simulink subsystem "Subsystem_Driver_Battery_BAv02"  (R2022b)
settings: Solver=VariableStepAuto  StartTime=0.0  StopTime=10.0  RelTol=1e-3
undefined symbols (not defined in the file): driver, param, route, weatherSim
libraries: slpidlib x3
settings Model: Creator=giaco  LastModifiedBy=giaco

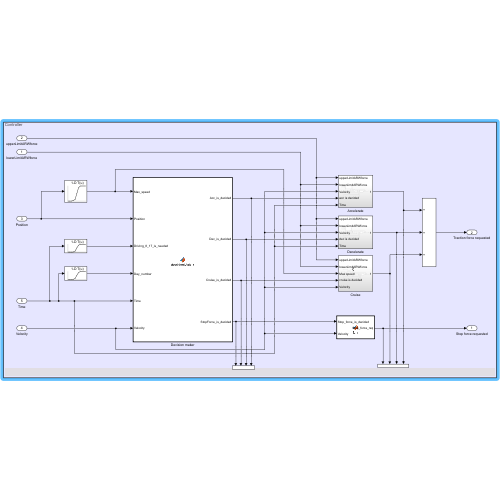
[thumbnail: Simulink's stored preview of the top-level diagram]
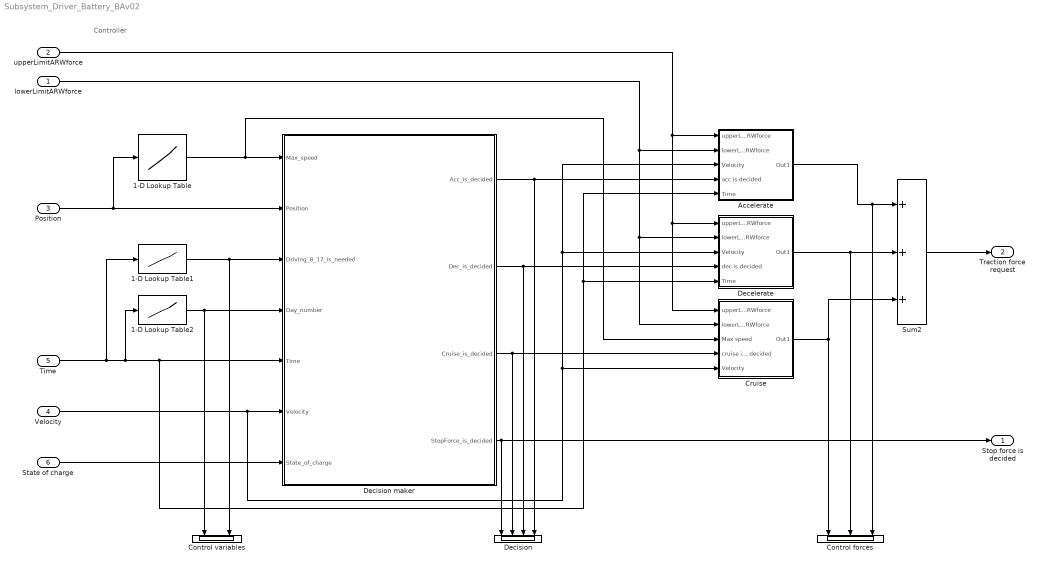
== system Subsystem_Driver_Battery_BAv02 ==
  note: Controller
  lowerLimitARWforce : Inport
  upperLimitARWforce : Inport  Port=2
  Position : Inport  Port=3
  Velocity : Inport  Port=4
  Time : Inport  Port=5
  State of charge : Inport  Port=6
  1-D Lookup Table : Lookup_n-D  NumberOfTableDimensions=1  BreakpointsForDimension1=route.dist  Table=route.maxSpeed  InternalRulePriority=Speed  RndMeth=Simplest
  1-D Lookup Table1 : Lookup_n-D  NumberOfTableDimensions=1  BreakpointsForDimension1=weatherSim.irradiance.timeSec  Table=weatherSim.irradiance.driving_8_17_Sec  InternalRulePriority=Speed
  1-D Lookup Table2 : Lookup_n-D  NumberOfTableDimensions=1  BreakpointsForDimension1=weatherSim.irradiance.timeSec  Table=weatherSim.irradiance.dayNumSec  InternalRulePriority=Speed
  Accelerate : Subsystem
  Control forces : Scope  NumInputPorts=3
  Control variables : Scope  NumInputPorts=2
  Cruise : Subsystem
  Decelerate : Subsystem
  Decision : Scope  NumInputPorts=4
  Decision maker : MATLAB Function  TreatAsAtomicUnit=on
  Sum2 : Sum  Inputs=+++
  Stop force is decided : Outport
  Traction force request : Outport  Port=2
  wires:
  Decision maker/4(StopForce_is_decided) -> Stop force is decided/1, Decision/1
  Accelerate/1(Out1) -> Control forces/3, Sum2/1
  upperLimitARWforce/1 -> Decelerate/1(upperLimitARWforce), Cruise/1(upperLimitARWforce), Accelerate/1(upperLimitARWforce)
  Sum2/1 -> Traction force request/1
  Velocity/1 -> Decision maker/6(Velocity), Accelerate/3(Velocity), Decelerate/3(Velocity), Cruise/5(Velocity)
  Decision maker/2(Dec_is_decided) -> Decision/3, Decelerate/4(dec is decided)
  Decision maker/1(Acc_is_decided) -> Accelerate/4(acc is decided), Decision/4
  lowerLimitARWforce/1 -> Accelerate/2(lowerLimitARWforce), Decelerate/2(lowerLimitARWforce), Cruise/2(lowerLimitARWforce)
  1-D Lookup Table/1 -> Decision maker/1(Max_speed), Cruise/3(Max speed)
  Decelerate/1(Out1) -> Control forces/2, Sum2/2
  Time/1 -> 1-D Lookup Table1/1, 1-D Lookup Table2/1, Decision maker/5(Time), Accelerate/5(Time), Decelerate/5(Time)
  Decision maker/3(Cruise_is_decided) -> Decision/2, Cruise/4(cruise is decided)
  Cruise/1(Out1) -> Control forces/1, Sum2/3
  Position/1 -> Decision maker/2(Position), 1-D Lookup Table/1
  1-D Lookup Table1/1 -> Control variables/2, Decision maker/3(Driving_8_17_is_needed)
  1-D Lookup Table2/1 -> Control variables/1, Decision maker/4(Day_number)
  State of charge/1 -> Decision maker/7(State_of_charge)

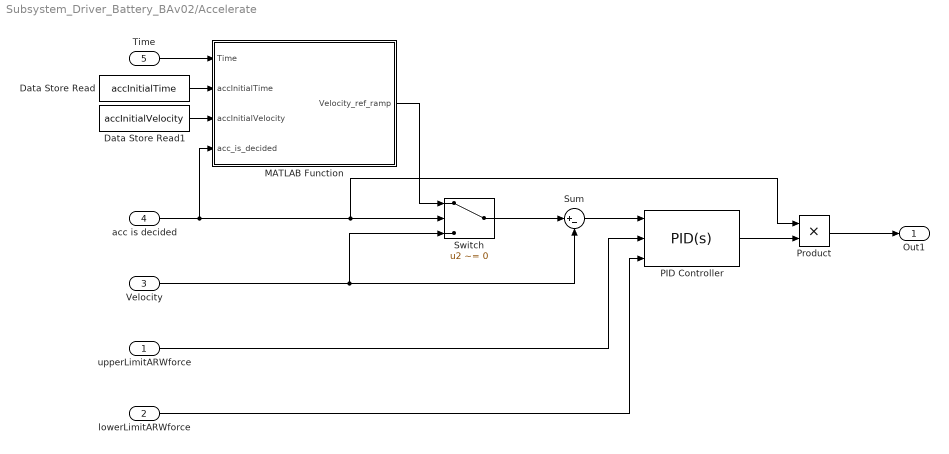
== system Subsystem_Driver_Battery_BAv02/Accelerate ==
  upperLimitARWforce : Inport
  lowerLimitARWforce : Inport  Port=2
  Velocity : Inport  Port=3
  acc is decided : Inport  Port=4
  Time : Inport  Port=5
  Data Store Read : DataStoreRead  DataStoreName=accInitialTime  IndexOptions=Index vector (dialog)  Indices=1  OutputSizes=1
  Data Store Read1 : DataStoreRead  DataStoreName=accInitialVelocity  IndexOptions=Index vector (dialog)  Indices=1  OutputSizes=1
  MATLAB Function : MATLAB Function  TreatAsAtomicUnit=on
  PID Controller : slpidlib/PID Controller  Controller=PID  Form=Ideal  TimeDomain=Continuous-time  UseExternalTs=off  SampleTime=-1  IntegratorMethod=Forward Euler  FilterMethod=Forward Euler  ControllerParametersSource=internal  P=4000  I=80/1  UseKiTs=off  D=0  N=100  UseFilter=on  TunerSelectOption=Transfer Function Based (PID Tuner App)  InitialConditionSource=internal  InitialConditionForIntegrator=0  InitialConditionForFilter=0  DifferentiatorICPrevScaledInput=0  ExternalReset=none  TrackingMode=off  Kt=1  LimitOutput=on  SatLimitsSource=external  UpperSaturationLimit=param.motor.maxTorque * param.motor.transmissionRatio / param.suspension.rWheel  LowerSaturationLimit=param.motor.minTorque * param.motor.transmissionRatio / param.suspension.rWheel  LinearizeAsGain=on  AntiWindupMode=none  Kb=1  LimitIntegrator=off  UpperIntegratorSaturationLimit=inf  LowerIntegratorSaturationLimit=-inf  POutMin=[]  POutMax=[]  IOutMin=[]  IOutMax=[]  DOutMin=[]  DOutMax=[]  NOutMin=[]  NOutMax=[]  SumOutMin=[]  SumOutMax=[]  SaturationOutMin=[]  SaturationOutMax=[]  PParamMin=[]  PParamMax=[]  IParamMin=[]  IParamMax=[]  DParamMin=[]  DParamMax=[]  NParamMin=[]  NParamMax=[]  KbParamMin=[]  KbParamMax=[]  KtParamMin=[]  KtParamMax=[]  KbOutMin=[]  KbOutMax=[]  KtOutMin=[]  KtOutMax=[]  IntegratorOutMin=[]  IntegratorOutMax=[]  FilterOutMin=[]  FilterOutMax=[]  SumI1OutMin=[]  SumI1OutMax=[]  SumI2OutMin=[]  SumI2OutMax=[]  SumI3OutMin=[]  SumI3OutMax=[]  SumI4OutMin=[]  SumI4OutMax=[]  SumDOutMin=[]  SumDOutMax=[]  DifferentiatorOutMin=[]  DifferentiatorOutMax=[]  FilterDiffOutCoefMin=[]  FilterDiffOutCoefMax=[]  ReciprocalOutMin=[]  ReciprocalOutMax=[]  SumDenOutMin=[]  SumDenOutMax=[]  SumNumOutMin=[]  SumNumOutMax=[]  DivideOutMin=[]  DivideOutMax=[]  UdiffTsProdOutMin=[]  UdiffTsProdOutMax=[]  NTsProdOutMin=[]  NTsProdOutMax=[]  UintegralTsProdOutMin=[]  UintegralTsProdOutMax=[]  UngainTsProdOutMin=[]  UngainTsProdOutMax=[]  ClampingZeroOutDataTypeStr=Inherit: Inherit via back propagation  ClampingZeroOutMin=[]  ClampingZeroOutMax=[]  FilterDenConstantOutDataTypeStr=Inherit: Inherit via back propagation  FilterDenConstantOutMin=[]  FilterDenConstantOutMax=[]  PCopyOutDataTypeStr=Inherit: Inherit via back propagation  PCopyOutMin=[]  PCopyOutMax=[]  NCopyOutDataTypeStr=Inherit: Inherit via back propagation  NCopyOutMin=[]  NCopyOutMax=[]  IntegratorContinuousStateAttributes=''  IntegratorStateMustResolveToSignalObject=off  IntegratorRTWStateStorageClass=Auto  FilterContinuousStateAttributes=''  FilterStateMustResolveToSignalObject=off  FilterRTWStateStorageClass=Auto  ParallelPVariant=Passthrough  IdealPVariant=InternalParameters  IVariant=InternalParameters  DVariant=InternalParameters  IntegratorVariant=Continuous  SatVariant=External  AWVariant=Passthrough  PCopyVariant=Disabled  TRVariant=Disabled  FdbkBlocksVariant=Forward  IdealPFdbkVariant=Disabled  SatFdbkVariant=Disabled  DerivativeFilterVariant=ContFilter  NVariant=InternalParameters  NCopyVariant=Disabled  FilterICVariant=InternalICsFilter  IntegratorICVariant=InternalICs  ExternalResetVariant=Disabled  TRSumVariant=Passthrough  SumFdbkVariant=Disabled  SumVariant=Sum_PID  TsampFilterVariant=InternalTs  TsampNgainVariant=Passthrough  TsampIntegralVariant=Passthrough  ExternalSaturationOutDataTypeStr=Inherit: Same as second input
  Product : Product
  Sum : Sum  Inputs=|+-
  Switch : Switch  Criteria=u2 ~= 0  SaturateOnIntegerOverflow=off  InputSameDT=off
  Out1 : Outport
  wires:
  acc is decided/1 -> MATLAB Function/4(acc_is_decided), Product/1, Switch/2
  Switch/1 -> Sum/1
  Velocity/1 -> Sum/2, Switch/3
  Sum/1 -> PID Controller/1
  PID Controller/1 -> Product/2
  Product/1 -> Out1/1
  Time/1 -> MATLAB Function/1(Time)
  MATLAB Function/1(Velocity_ref_ramp) -> Switch/1
  Data Store Read/1 -> MATLAB Function/2(accInitialTime)
  Data Store Read1/1 -> MATLAB Function/3(accInitialVelocity)
  upperLimitARWforce/1 -> PID Controller/2
  lowerLimitARWforce/1 -> PID Controller/3

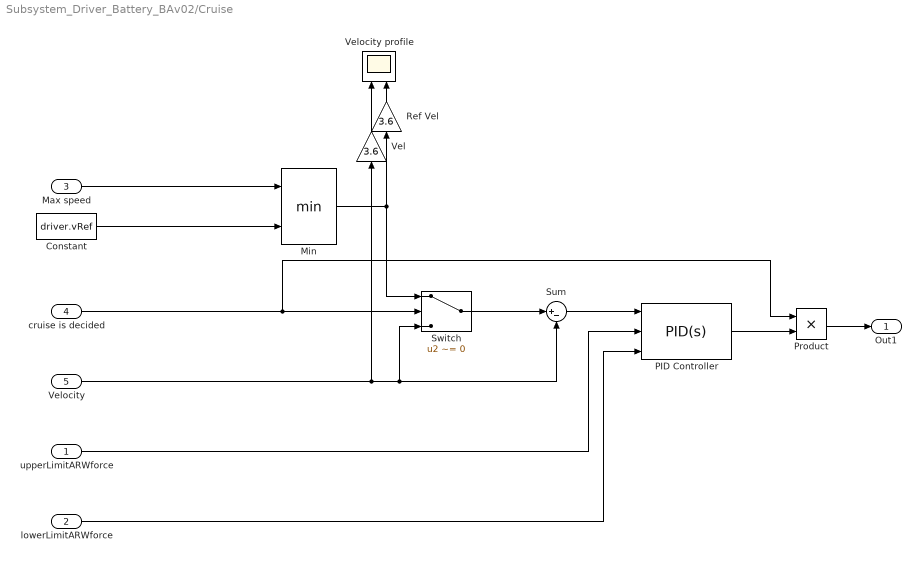
== system Subsystem_Driver_Battery_BAv02/Cruise ==
  upperLimitARWforce : Inport
  lowerLimitARWforce : Inport  Port=2
  Max speed : Inport  Port=3
  cruise is decided : Inport  Port=4
  Velocity : Inport  Port=5
  Constant : Constant  Value=driver.vRef
  Min : MinMax  Inputs=2
  PID Controller : slpidlib/PID Controller  Controller=PID  Form=Ideal  TimeDomain=Continuous-time  UseExternalTs=off  SampleTime=-1  IntegratorMethod=Forward Euler  FilterMethod=Forward Euler  ControllerParametersSource=internal  P=2000  I=1/500  UseKiTs=off  D=0  N=100  UseFilter=on  TunerSelectOption=Transfer Function Based (PID Tuner App)  InitialConditionSource=internal  InitialConditionForIntegrator=0  InitialConditionForFilter=0  DifferentiatorICPrevScaledInput=0  ExternalReset=none  TrackingMode=off  Kt=1  LimitOutput=on  SatLimitsSource=external  UpperSaturationLimit=param.motor.maxTorque * param.motor.transmissionRatio / param.suspension.rWheel  LowerSaturationLimit=param.motor.minTorque * param.motor.transmissionRatio / param.suspension.rWheel  LinearizeAsGain=on  AntiWindupMode=none  Kb=1  LimitIntegrator=off  UpperIntegratorSaturationLimit=inf  LowerIntegratorSaturationLimit=-inf  POutMin=[]  POutMax=[]  IOutMin=[]  IOutMax=[]  DOutMin=[]  DOutMax=[]  NOutMin=[]  NOutMax=[]  SumOutMin=[]  SumOutMax=[]  SaturationOutMin=[]  SaturationOutMax=[]  PParamMin=[]  PParamMax=[]  IParamMin=[]  IParamMax=[]  DParamMin=[]  DParamMax=[]  NParamMin=[]  NParamMax=[]  KbParamMin=[]  KbParamMax=[]  KtParamMin=[]  KtParamMax=[]  KbOutMin=[]  KbOutMax=[]  KtOutMin=[]  KtOutMax=[]  IntegratorOutMin=[]  IntegratorOutMax=[]  FilterOutMin=[]  FilterOutMax=[]  SumI1OutMin=[]  SumI1OutMax=[]  SumI2OutMin=[]  SumI2OutMax=[]  SumI3OutMin=[]  SumI3OutMax=[]  SumI4OutMin=[]  SumI4OutMax=[]  SumDOutMin=[]  SumDOutMax=[]  DifferentiatorOutMin=[]  DifferentiatorOutMax=[]  FilterDiffOutCoefMin=[]  FilterDiffOutCoefMax=[]  ReciprocalOutMin=[]  ReciprocalOutMax=[]  SumDenOutMin=[]  SumDenOutMax=[]  SumNumOutMin=[]  SumNumOutMax=[]  DivideOutMin=[]  DivideOutMax=[]  UdiffTsProdOutMin=[]  UdiffTsProdOutMax=[]  NTsProdOutMin=[]  NTsProdOutMax=[]  UintegralTsProdOutMin=[]  UintegralTsProdOutMax=[]  UngainTsProdOutMin=[]  UngainTsProdOutMax=[]  ClampingZeroOutDataTypeStr=Inherit: Inherit via back propagation  ClampingZeroOutMin=[]  ClampingZeroOutMax=[]  FilterDenConstantOutDataTypeStr=Inherit: Inherit via back propagation  FilterDenConstantOutMin=[]  FilterDenConstantOutMax=[]  PCopyOutDataTypeStr=Inherit: Inherit via back propagation  PCopyOutMin=[]  PCopyOutMax=[]  NCopyOutDataTypeStr=Inherit: Inherit via back propagation  NCopyOutMin=[]  NCopyOutMax=[]  IntegratorContinuousStateAttributes=''  IntegratorStateMustResolveToSignalObject=off  IntegratorRTWStateStorageClass=Auto  FilterContinuousStateAttributes=''  FilterStateMustResolveToSignalObject=off  FilterRTWStateStorageClass=Auto  ParallelPVariant=Passthrough  IdealPVariant=InternalParameters  IVariant=InternalParameters  DVariant=InternalParameters  IntegratorVariant=Continuous  SatVariant=External  AWVariant=Passthrough  PCopyVariant=Disabled  TRVariant=Disabled  FdbkBlocksVariant=Forward  IdealPFdbkVariant=Disabled  SatFdbkVariant=Disabled  DerivativeFilterVariant=ContFilter  NVariant=InternalParameters  NCopyVariant=Disabled  FilterICVariant=InternalICsFilter  IntegratorICVariant=InternalICs  ExternalResetVariant=Disabled  TRSumVariant=Passthrough  SumFdbkVariant=Disabled  SumVariant=Sum_PID  TsampFilterVariant=InternalTs  TsampNgainVariant=Passthrough  TsampIntegralVariant=Passthrough  ExternalSaturationOutDataTypeStr=Inherit: Same as second input
  Product : Product
  Ref Vel : Gain  Gain=3.6
  Sum : Sum  Inputs=|+-
  Switch : Switch  Criteria=u2 ~= 0  SaturateOnIntegerOverflow=off  InputSameDT=off
  Vel : Gain  Gain=3.6
  Velocity profile : Scope  NumInputPorts=2
  Out1 : Outport
  wires:
  cruise is decided/1 -> Product/1, Switch/2
  Max speed/1 -> Min/1
  Constant/1 -> Min/2
  Velocity/1 -> Vel/1, Switch/3, Sum/2
  Switch/1 -> Sum/1
  PID Controller/1 -> Product/2
  Sum/1 -> PID Controller/1
  Product/1 -> Out1/1
  lowerLimitARWforce/1 -> PID Controller/3
  upperLimitARWforce/1 -> PID Controller/2
  Ref Vel/1 -> Velocity profile/2
  Min/1 -> Switch/1, Ref Vel/1
  Vel/1 -> Velocity profile/1

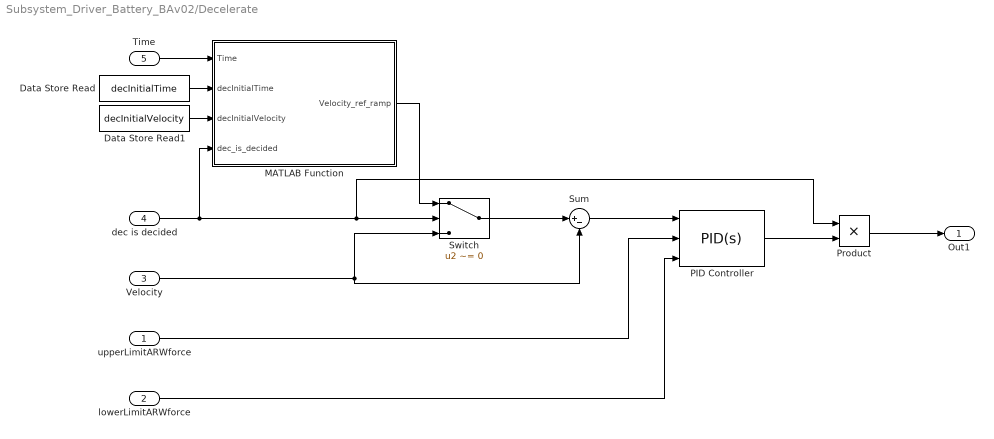
== system Subsystem_Driver_Battery_BAv02/Decelerate ==
  upperLimitARWforce : Inport
  lowerLimitARWforce : Inport  Port=2
  Velocity : Inport  Port=3
  dec is decided : Inport  Port=4
  Time : Inport  Port=5
  Data Store Read : DataStoreRead  DataStoreName=decInitialTime  IndexOptions=Index vector (dialog)  Indices=1  OutputSizes=1
  Data Store Read1 : DataStoreRead  DataStoreName=decInitialVelocity  IndexOptions=Index vector (dialog)  Indices=1  OutputSizes=1
  MATLAB Function : MATLAB Function  TreatAsAtomicUnit=on
  PID Controller : slpidlib/PID Controller  Controller=PID  Form=Ideal  TimeDomain=Continuous-time  UseExternalTs=off  SampleTime=-1  IntegratorMethod=Forward Euler  FilterMethod=Forward Euler  ControllerParametersSource=internal  P=4000  I=1/1  UseKiTs=off  D=0  N=100  UseFilter=on  TunerSelectOption=Transfer Function Based (PID Tuner App)  InitialConditionSource=internal  InitialConditionForIntegrator=0  InitialConditionForFilter=0  DifferentiatorICPrevScaledInput=0  ExternalReset=none  TrackingMode=off  Kt=1  LimitOutput=on  SatLimitsSource=external  UpperSaturationLimit=param.motor.maxTorque * param.motor.transmissionRatio / param.suspension.rWheel  LowerSaturationLimit=param.motor.minTorque * param.motor.transmissionRatio / param.suspension.rWheel  LinearizeAsGain=on  AntiWindupMode=none  Kb=1  LimitIntegrator=off  UpperIntegratorSaturationLimit=inf  LowerIntegratorSaturationLimit=-inf  POutMin=[]  POutMax=[]  IOutMin=[]  IOutMax=[]  DOutMin=[]  DOutMax=[]  NOutMin=[]  NOutMax=[]  SumOutMin=[]  SumOutMax=[]  SaturationOutMin=[]  SaturationOutMax=[]  PParamMin=[]  PParamMax=[]  IParamMin=[]  IParamMax=[]  DParamMin=[]  DParamMax=[]  NParamMin=[]  NParamMax=[]  KbParamMin=[]  KbParamMax=[]  KtParamMin=[]  KtParamMax=[]  KbOutMin=[]  KbOutMax=[]  KtOutMin=[]  KtOutMax=[]  IntegratorOutMin=[]  IntegratorOutMax=[]  FilterOutMin=[]  FilterOutMax=[]  SumI1OutMin=[]  SumI1OutMax=[]  SumI2OutMin=[]  SumI2OutMax=[]  SumI3OutMin=[]  SumI3OutMax=[]  SumI4OutMin=[]  SumI4OutMax=[]  SumDOutMin=[]  SumDOutMax=[]  DifferentiatorOutMin=[]  DifferentiatorOutMax=[]  FilterDiffOutCoefMin=[]  FilterDiffOutCoefMax=[]  ReciprocalOutMin=[]  ReciprocalOutMax=[]  SumDenOutMin=[]  SumDenOutMax=[]  SumNumOutMin=[]  SumNumOutMax=[]  DivideOutMin=[]  DivideOutMax=[]  UdiffTsProdOutMin=[]  UdiffTsProdOutMax=[]  NTsProdOutMin=[]  NTsProdOutMax=[]  UintegralTsProdOutMin=[]  UintegralTsProdOutMax=[]  UngainTsProdOutMin=[]  UngainTsProdOutMax=[]  ClampingZeroOutDataTypeStr=Inherit: Inherit via back propagation  ClampingZeroOutMin=[]  ClampingZeroOutMax=[]  FilterDenConstantOutDataTypeStr=Inherit: Inherit via back propagation  FilterDenConstantOutMin=[]  FilterDenConstantOutMax=[]  PCopyOutDataTypeStr=Inherit: Inherit via back propagation  PCopyOutMin=[]  PCopyOutMax=[]  NCopyOutDataTypeStr=Inherit: Inherit via back propagation  NCopyOutMin=[]  NCopyOutMax=[]  IntegratorContinuousStateAttributes=''  IntegratorStateMustResolveToSignalObject=off  IntegratorRTWStateStorageClass=Auto  FilterContinuousStateAttributes=''  FilterStateMustResolveToSignalObject=off  FilterRTWStateStorageClass=Auto  ParallelPVariant=Passthrough  IdealPVariant=InternalParameters  IVariant=InternalParameters  DVariant=InternalParameters  IntegratorVariant=Continuous  SatVariant=External  AWVariant=Passthrough  PCopyVariant=Disabled  TRVariant=Disabled  FdbkBlocksVariant=Forward  IdealPFdbkVariant=Disabled  SatFdbkVariant=Disabled  DerivativeFilterVariant=ContFilter  NVariant=InternalParameters  NCopyVariant=Disabled  FilterICVariant=InternalICsFilter  IntegratorICVariant=InternalICs  ExternalResetVariant=Disabled  TRSumVariant=Passthrough  SumFdbkVariant=Disabled  SumVariant=Sum_PID  TsampFilterVariant=InternalTs  TsampNgainVariant=Passthrough  TsampIntegralVariant=Passthrough  ExternalSaturationOutDataTypeStr=Inherit: Same as second input
  Product : Product
  Sum : Sum  Inputs=|+-
  Switch : Switch  Criteria=u2 ~= 0  SaturateOnIntegerOverflow=off  InputSameDT=off
  Out1 : Outport
  wires:
  dec is decided/1 -> MATLAB Function/4(dec_is_decided), Product/1, Switch/2
  Switch/1 -> Sum/1
  Velocity/1 -> Sum/2, Switch/3
  PID Controller/1 -> Product/2
  Sum/1 -> PID Controller/1
  Product/1 -> Out1/1
  Time/1 -> MATLAB Function/1(Time)
  Data Store Read1/1 -> MATLAB Function/3(decInitialVelocity)
  MATLAB Function/1(Velocity_ref_ramp) -> Switch/1
  Data Store Read/1 -> MATLAB Function/2(decInitialTime)
  upperLimitARWforce/1 -> PID Controller/2
  lowerLimitARWforce/1 -> PID Controller/3

== matlab function Subsystem_Driver_Battery_BAv02/Accelerate/MATLAB Function ==
  data: Time input; Velocity_ref_ramp output; accInitialTime input; accInitialVelocity input; driver parameter; acc_is_decided input
function Velocity_ref_ramp = fcn(Time, accInitialTime, accInitialVelocity, driver, acc_is_decided)

Velocity_ref_ramp = 0;

if acc_is_decided
    Velocity_ref_ramp = driver.accRef .* (Time - accInitialTime) + accInitialVelocity;
end

== matlab function Subsystem_Driver_Battery_BAv02/Decelerate/MATLAB Function ==
  data: Time input; Velocity_ref_ramp output; decInitialTime input; decInitialVelocity input; driver parameter; dec_is_decided input
function Velocity_ref_ramp = fcn(Time, decInitialTime, decInitialVelocity, driver, dec_is_decided)

Velocity_ref_ramp = 0;

if dec_is_decided
    Velocity_ref_ramp = driver.decRef .* (Time - decInitialTime) + decInitialVelocity;
end

== matlab function Subsystem_Driver_Battery_BAv02/Decision maker ==
  settings: updateMethod=DISCRETE
  data: Max_speed input; Position input; Driving_8_17_is_needed input; Day_number input; Time input; Velocity input; spaceStopIsOver data_store_memory; timeStopIsNeeded data_store_memory; spaceStopIsNeeded data_store_memory; driver parameter; spaceStopNumber data_store_memory; spaceStopIsStarted data_store_memory; Acc_is_decided output; Dec_is_decided output; Cruise_is_decided output; StopForce_is_decided output; spaceStopInitialTime data_store_memory; accInitialTime data_store_memory; accInitialVelocity data_store_memory; decInitialTime data_store_memory; decInitialVelocity data_store_memory; racingDayIsStarted data_store_memory; dayNumber data_store_memory; weatherSim parameter; State_of_charge input; batteryIsEmpty data_store_memory; batteryStopIsOver data_store_memory
function [Acc_is_decided, Dec_is_decided, Cruise_is_decided, StopForce_is_decided] = decisionMaker(Max_speed, Position, Driving_8_17_is_needed, Day_number, Time, Velocity, driver, weatherSim, State_of_charge)

global racingDayIsStarted
global timeStopIsNeeded
global dayNumber

global spaceStopIsNeeded
global spaceStopIsStarted
global spaceStopIsOver
global spaceStopInitialTime
global spaceStopNumber

global batteryIsEmpty
global batteryStopIsOver

global accInitialTime
global accInitialVelocity
global decInitialTime
global decInitialVelocity

Acc_is_decided = false;
Dec_is_decided = false;
Cruise_is_decided = false;
StopForce_is_decided = false;

controlVelocity = min(driver.vRef, Max_speed);

%% Check for stops
% Time stops
stopTime = Time - Velocity ./ driver.decRef;

if ~timeStopIsNeeded && stopTime >= (weatherSim.irradiance.stopTimeSec(Day_number) - 60) %to be sure to stop on time
    timeStopIsNeeded = true;
    decInitialTime = Time; %initialization of time and velocity for ramp controller
    decInitialVelocity = Velocity;
end % if

% Space stops
stopDistance = Position - Velocity.^2 / (2 * driver.decRef);

if ~spaceStopIsNeeded && stopDistance >= driver.stopLocDist(spaceStopNumber)
    spaceStopIsNeeded = true;
    decInitialTime = Time; %initialization of time and velocity for ramp controller
    decInitialVelocity = Velocity;
    spaceStopNumber = spaceStopNumber + 1;
end % if

% Empty battery stops
if ~batteryIsEmpty && State_of_charge < 0.1
    batteryIsEmpty = true;
%     decInitialTime = Time; %initialization of time and velocity for ramp controller
%     decInitialVelocity = Velocity;
end % if

%% Check for new racing day
if Driving_8_17_is_needed && Day_number == dayNumber
    racingDayIsStarted = true;
    timeStopIsNeeded = false;
    dayNumber = dayNumber + 1;
end % if

%% Select control options
%% Deceleration
if timeStopIsNeeded
    if Velocity > driver.vRefStop
        Dec_is_decided = true;
    else %if Velocity <= driver.vRefStop
        StopForce_is_decided = true;
        Dec_is_decided = false;
    end % if

elseif batteryIsEmpty
    if Velocity > driver.vRefStop
        Dec_is_decided = true;
    else %if Velocity <= driver.vRefStop
        StopForce_is_decided = true;
        Dec_is_decided = false;
    end % if

    if State_of_charge > 0.3
        batteryIsEmpty = false;
        batteryStopIsOver = true;
    end % if

elseif spaceStopIsNeeded
    if spaceStopIsStarted
        spaceStopDuration = Time - spaceStopInitialTime;
        if spaceStopDuration >= 30*60
            spaceStopIsNeeded = false;
            spaceStopIsStarted = false;
            spaceStopIsOver = true;
            Acc_is_decided = true;
            accInitialTime = Time;
            accInitialVelocity = Velocity;
        else
            StopForce_is_decided = true;
        end % if
    else
        if Velocity > driver.vRefStop
            Dec_is_decided = true;
        else %if Velocity <= driver.vRefStop
            spaceStopIsStarted = true;
            spaceStopInitialTime = Time;
            StopForce_is_decided = true;
        end % if
    end % if

%% Acceleration
elseif racingDayIsStarted
    if Velocity < 0.9 * controlVelocity
        Acc_is_decided = true;
    else %if Velocity >= 0.9 * controlVelocity
        Cruise_is_decided = true;
        racingDayIsStarted = false;
    end % if

elseif spaceStopIsOver
    if Velocity < 0.9 * controlVelocity
        Acc_is_decided = true;
    else %if Velocity >= 0.9 * controlVelocity
        Cruise_is_decided = true;
        spaceStopIsOver = false;
    end % if
    
elseif batteryStopIsOver
    if Velocity < 0.9 * controlVelocity
        Acc_is_decided = true;
    else %if Velocity >= 0.9 * controlVelocity
        Cruise_is_decided = true;
        batteryStopIsOver = false;
    end % if

else
    Cruise_is_decided = true;
end % if
